simulink model "SwitchOneIR(1)"  (R2019a)
settings: Solver=FixedStepAuto  StartTime=0.0  StopTime=10.0  RelTol=1e-3
libraries: vexarmcortexlib x23, vexcommonlib x3
settings Model: ExtModeTrigDuration=25  Creator=hsstudent  LastModifiedBy=hsstudent
settings SolverCC: AutoInsertRateTranBlk=on
settings OptimizationCC: EnhancedBackFolding=on  PassReuseOutputArgsAs=Individual arguments  MaxStackSize=64  OptimizeBlockOrder=speed  DifferentSizesBufferReuse=on  OptimizationCustomize=off
settings DebuggingCC: ParameterTunabilityLossMsg=error
settings HardwareCC: ProdBitPerPointer=32  ProdBitPerSizeT=32  ProdBitPerPtrDiffT=32  ProdLargestAtomicInteger=Long  ProdLargestAtomicFloat=Double  ProdWordSize=32  ProdHWDeviceType=ARM Compatible->ARM Cortex
settings SFSimCC: MATLABDynamicMemAlloc=off
settings RTWCC: SystemTargetFile=ert.tlc  HardwareBoard=ARM Cortex-based VEX Microcontroller  TLCOptions="-aInlineSetEventsForThisBaseRateFcn=TLC_FALSE -aSuppressMultiTaskScheduler=TLC_FALSE  -aRateBasedStepFcn=0"  TemplateMakefile=ert_default_tmf  GenerateReport=on  Toolchain=GNU Tools for VEX ARM Cortex  IncludeHyperlinkInReport=on  LaunchReport=on  GenerateTraceInfo=on  GenerateTraceReport=on  GenerateTraceReportSl=on  GenerateTraceReportSf=on  GenerateTraceReportEml=on
settings CodeAppCC: ForceParamTrailComments=on  IgnoreCustomStorageClasses=off  OperatorAnnotations=on  SimulinkDataObjDesc=on  SFDataObjDesc=on  InsertBlockDesc=on

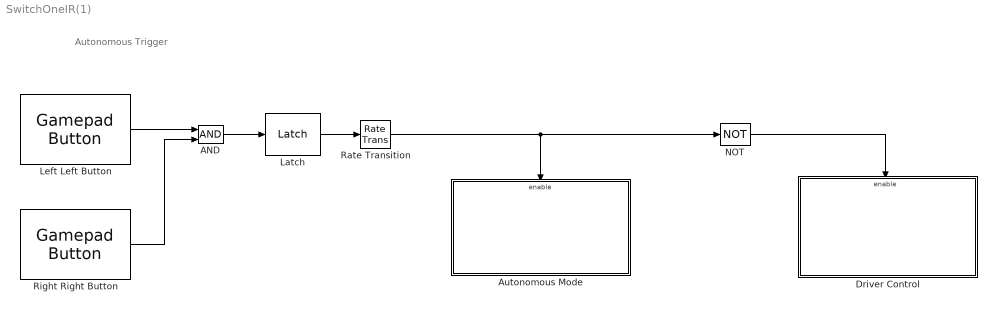
== system SwitchOneIR(1) ==
  note: Autonomous Trigger
  AND : Logic  IconShape=distinctive  AllPortsSameDT=off  OutDataTypeStr=boolean
  Autonomous Mode : Subsystem
  Driver Control : Subsystem  TreatAsAtomicUnit=on
  Latch : vexcommonlib/Latch  output0=off  BlockPlatform=vexarmcortex
      settings: SourceProductName=Simulink Coder Support Package for ARM Cortex-based VEX Microcontroller  SourceProductBaseCode=EC_VEX_MICRO
  Left Left Button : vexarmcortexlib/Gamepad/Gamepad Button  joystick=1  chan=7  button56=Down  button78=Left  SimulationIn=off  SampleTime=0.5
      settings: SourceProductName=Simulink Coder Support Package for ARM Cortex-based VEX Microcontroller  SourceProductBaseCode=EC_VEX_MICRO
  NOT : Logic  Operator=NOT  IconShape=distinctive  AllPortsSameDT=off  OutDataTypeStr=boolean
  Rate Transition : RateTransition
  Right Right Button : vexarmcortexlib/Gamepad/Gamepad Button  joystick=1  chan=8  button56=Down  button78=Right  SimulationIn=off  SampleTime=0.5
      settings: SourceProductName=Simulink Coder Support Package for ARM Cortex-based VEX Microcontroller  SourceProductBaseCode=EC_VEX_MICRO
  wires:
  Rate Transition/1 -> NOT/1, Autonomous Mode/Enable
  AND/1 -> Latch/1
  NOT/1 -> Driver Control/Enable
  Left Left Button/1 -> AND/1
  Latch/1 -> Rate Transition/1
  Right Right Button/1 -> AND/2

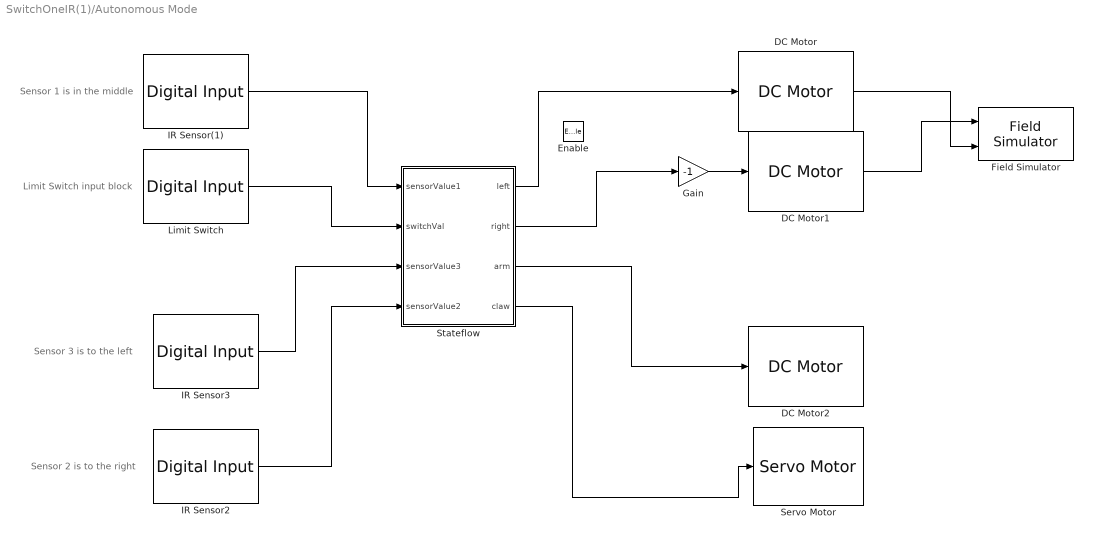
== system SwitchOneIR(1)/Autonomous Mode ==
  note: Sensor 2 is to the right
  note: Sensor 1 is in the middle
  note: Limit Switch input block
  note: Sensor 3 is to the left
  Enable : EnablePort  StatesWhenEnabling=reset
  DC Motor : vexarmcortexlib/Actuators/DC Motor  motor=6  scaleFactor=1/13.5  SimulationOut=on
      settings: SourceProductName=Simulink Coder Support Package for ARM Cortex-based VEX Microcontroller  SourceProductBaseCode=EC_VEX_MICRO
  DC Motor1 : vexarmcortexlib/Actuators/DC Motor  motor=2  scaleFactor=1/13.5  SimulationOut=on
      settings: SourceProductName=Simulink Coder Support Package for ARM Cortex-based VEX Microcontroller  SourceProductBaseCode=EC_VEX_MICRO
  DC Motor2 : vexarmcortexlib/Actuators/DC Motor  motor=9  scaleFactor=1/13.5  SimulationOut=off
      settings: SourceProductName=Simulink Coder Support Package for ARM Cortex-based VEX Microcontroller  SourceProductBaseCode=EC_VEX_MICRO
  Field Simulator : vexcommonlib/Field Simulator  radius=2.5  space=10  range=200  BlockPlatform=vexarmcortex
      settings: SourceProductName=Simulink Coder Support Package for ARM Cortex-based VEX Microcontroller  SourceProductBaseCode=EC_VEX_MICRO
  Gain : Gain  Gain=-1
  IR Sensor(1) : vexarmcortexlib/Sensors/Digital Input  inChan=2  SimulationIn=off  SampleTime=0.05
      settings: SourceProductName=Simulink Coder Support Package for ARM Cortex-based VEX Microcontroller  SourceProductBaseCode=EC_VEX_MICRO
  IR Sensor2 : vexarmcortexlib/Sensors/Digital Input  inChan=8  SimulationIn=off  SampleTime=0.05
      settings: SourceProductName=Simulink Coder Support Package for ARM Cortex-based VEX Microcontroller  SourceProductBaseCode=EC_VEX_MICRO
  IR Sensor3 : vexarmcortexlib/Sensors/Digital Input  inChan=5  SimulationIn=off  SampleTime=0.05
      settings: SourceProductName=Simulink Coder Support Package for ARM Cortex-based VEX Microcontroller  SourceProductBaseCode=EC_VEX_MICRO
  Limit Switch : vexarmcortexlib/Sensors/Digital Input  inChan=6  SimulationIn=off  SampleTime=0.05
      settings: SourceProductName=Simulink Coder Support Package for ARM Cortex-based VEX Microcontroller  SourceProductBaseCode=EC_VEX_MICRO
  Servo Motor : vexarmcortexlib/Actuators/Servo Motor  motor=3  scaleFactor=60/127  SimulationOut=off
      settings: SourceProductName=Simulink Coder Support Package for ARM Cortex-based VEX Microcontroller  SourceProductBaseCode=EC_VEX_MICRO
  Stateflow : Stateflow chart  TreatAsAtomicUnit=on
  wires:
  DC Motor/1 -> Field Simulator/2
  Gain/1 -> DC Motor1/1
  DC Motor1/1 -> Field Simulator/1
  Stateflow/1(left) -> DC Motor/1
  Stateflow/2(right) -> Gain/1
  IR Sensor(1)/1 -> Stateflow/1(sensorValue1)
  Limit Switch/1 -> Stateflow/2(switchVal)
  Stateflow/3(arm) -> DC Motor2/1
  Stateflow/4(claw) -> Servo Motor/1
  IR Sensor2/1 -> Stateflow/4(sensorValue2)
  IR Sensor3/1 -> Stateflow/3(sensorValue3)

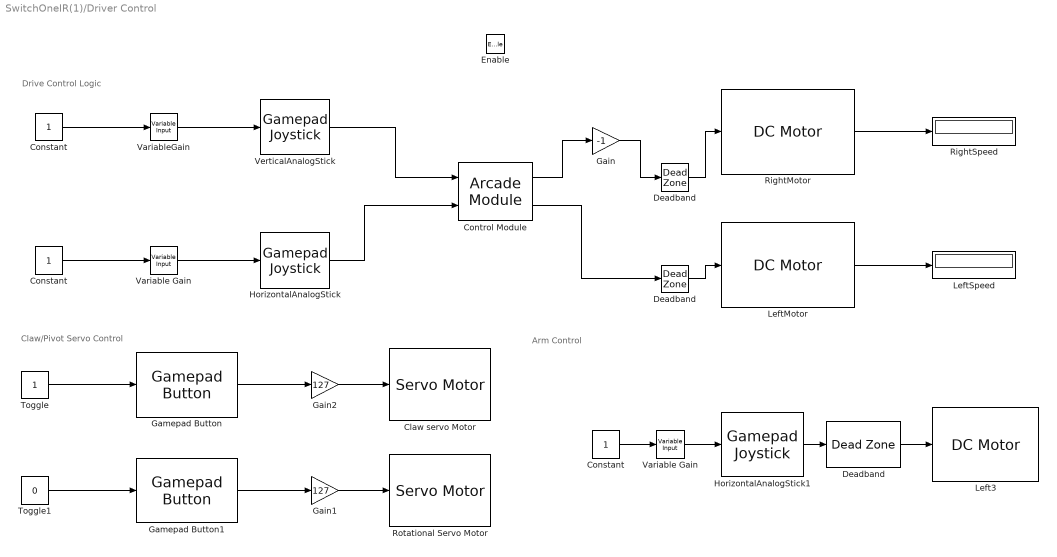
== system SwitchOneIR(1)/Driver Control ==
  note: Claw/Pivot Servo Control
  note: Drive Control Logic
  note: Arm Control
  Enable : EnablePort  StatesWhenEnabling=reset
  "  Deadband " : DeadZone  LowerValue=-30  UpperValue=30  SaturateOnIntegerOverflow=on
  " Constant " : Constant
  " Variable Gain " : vexarmcortexlib/Utilities/Variable Input  low=-127  gain=-68  high=127
      settings: SourceProductName=Simulink Coder Support Package for ARM Cortex-based VEX Microcontroller  SourceProductBaseCode=EC_VEX_MICRO
  Claw servo Motor : vexarmcortexlib/Actuators/Servo Motor  motor=3  scaleFactor=60/127  SimulationOut=off
      settings: SourceProductName=Simulink Coder Support Package for ARM Cortex-based VEX Microcontroller  SourceProductBaseCode=EC_VEX_MICRO
  Constant : Constant
  "Constant " : Constant
  Control Module : vexcommonlib/Arcade Module  BlockPlatform=vexarmcortex
      settings: SourceProductName=Simulink Coder Support Package for ARM Cortex-based VEX Microcontroller  SourceProductBaseCode=EC_VEX_MICRO
  Deadband : DeadZone  SaturateOnIntegerOverflow=on
  "Deadband " : DeadZone  LowerValue=-30  UpperValue=30  SaturateOnIntegerOverflow=on
  Gain : Gain  Gain=-1
  Gain1 : Gain  Gain=127
  Gain2 : Gain  Gain=127
  Gamepad Button : vexarmcortexlib/Gamepad/Gamepad Button  joystick=1  chan=6  button56=Down  button78=Down  SimulationIn=on  SampleTime=0.02
      settings: SourceProductName=Simulink Coder Support Package for ARM Cortex-based VEX Microcontroller  SourceProductBaseCode=EC_VEX_MICRO
  Gamepad Button1 : vexarmcortexlib/Gamepad/Gamepad Button  joystick=1  chan=5  button56=Up  button78=Down  SimulationIn=on  SampleTime=0.02
      settings: SourceProductName=Simulink Coder Support Package for ARM Cortex-based VEX Microcontroller  SourceProductBaseCode=EC_VEX_MICRO
  HorizontalAnalogStick : vexarmcortexlib/Gamepad/Gamepad Joystick  joystick=1  chan=1  SimulationIn=on  SampleTime=0.02
      settings: SourceProductName=Simulink Coder Support Package for ARM Cortex-based VEX Microcontroller  SourceProductBaseCode=EC_VEX_MICRO
  HorizontalAnalogStick1 : vexarmcortexlib/Gamepad/Gamepad Joystick  joystick=1  chan=3  SimulationIn=on  SampleTime=0.02
      settings: SourceProductName=Simulink Coder Support Package for ARM Cortex-based VEX Microcontroller  SourceProductBaseCode=EC_VEX_MICRO
  Left3 : vexarmcortexlib/Actuators/DC Motor  motor=9  scaleFactor=1/13.5  SimulationOut=off
      settings: SourceProductName=Simulink Coder Support Package for ARM Cortex-based VEX Microcontroller  SourceProductBaseCode=EC_VEX_MICRO
  LeftMotor : vexarmcortexlib/Actuators/DC Motor  motor=6  scaleFactor=1/13.5  SimulationOut=on
      settings: SourceProductName=Simulink Coder Support Package for ARM Cortex-based VEX Microcontroller  SourceProductBaseCode=EC_VEX_MICRO
  LeftSpeed : Display
  RightMotor : vexarmcortexlib/Actuators/DC Motor  motor=2  scaleFactor=1/13.5  SimulationOut=on
      settings: SourceProductName=Simulink Coder Support Package for ARM Cortex-based VEX Microcontroller  SourceProductBaseCode=EC_VEX_MICRO
  RightSpeed : Display
  "Rotational Servo Motor " : vexarmcortexlib/Actuators/Servo Motor  motor=8  scaleFactor=60/127  SimulationOut=off
      settings: SourceProductName=Simulink Coder Support Package for ARM Cortex-based VEX Microcontroller  SourceProductBaseCode=EC_VEX_MICRO
  Toggle : Constant
      settings: OpenFcn=|
      | if strcmp('0',get_param(gcb, 'Value'))                        set_param(gcb, 'Value', '1');
      | else
      |             set_param(gcb, 'Value', '0');
      | end
  Toggle1 : Constant  Value=0
      settings: OpenFcn=|
      | if strcmp('0',get_param(gcb, 'Value'))                        set_param(gcb, 'Value', '1');
      | else
      |             set_param(gcb, 'Value', '0');
      | end
  Variable Gain : vexarmcortexlib/Utilities/Variable Input  low=-127  gain=-118.8065  high=127
      settings: SourceProductName=Simulink Coder Support Package for ARM Cortex-based VEX Microcontroller  SourceProductBaseCode=EC_VEX_MICRO
  "VariableGain " : vexarmcortexlib/Utilities/Variable Input  low=-127  gain=0  high=127
      settings: SourceProductName=Simulink Coder Support Package for ARM Cortex-based VEX Microcontroller  SourceProductBaseCode=EC_VEX_MICRO
  VerticalAnalogStick : vexarmcortexlib/Gamepad/Gamepad Joystick  joystick=1  chan=2  SimulationIn=on  SampleTime=0.02
      settings: SourceProductName=Simulink Coder Support Package for ARM Cortex-based VEX Microcontroller  SourceProductBaseCode=EC_VEX_MICRO
  wires:
  Gain2/1 -> Claw servo Motor/1
  Toggle/1 -> Gamepad Button/1
  "Deadband "/1 -> RightMotor/1
  " Variable Gain "/1 -> HorizontalAnalogStick1/1
  " Constant "/1 -> " Variable Gain "/1
  "  Deadband "/1 -> LeftMotor/1
  HorizontalAnalogStick1/1 -> Deadband/1
  Control Module/1 -> Gain/1
  Constant/1 -> "VariableGain "/1
  "VariableGain "/1 -> VerticalAnalogStick/1
  RightMotor/1 -> RightSpeed/1
  Variable Gain/1 -> HorizontalAnalogStick/1
  LeftMotor/1 -> LeftSpeed/1
  Control Module/2 -> "  Deadband "/1
  "Constant "/1 -> Variable Gain/1
  Gamepad Button/1 -> Gain2/1
  Gain/1 -> "Deadband "/1
  VerticalAnalogStick/1 -> Control Module/1
  HorizontalAnalogStick/1 -> Control Module/2
  Deadband/1 -> Left3/1
  Toggle1/1 -> Gamepad Button1/1
  Gain1/1 -> "Rotational Servo Motor "/1
  Gamepad Button1/1 -> Gain1/1

== stateflow chart SwitchOneIR(1)/Autonomous Mode/Stateflow ==
  state Stop
    entry:
    left = 0;
    right= 0;
  state GoForward
    entry:
    left = 100;
    right = 100;
  state GoLeft
    entry:
    left = -50
    right = 50
  note: 
  state Drop
    entry:
    arm = -25;
    left = 0;
    right = 0;
  state GoRight
    entry:
    left = 50
    right = -50
  state ClawDrop
    entry:
    claw = 127;
    left = 0;
    right = 0;
    arm = 0;
  state TowerDetect
    entry:
    left = 0;
    right = 0;
  state Stop2
    entry:
    arm = 0;
    left = 0;
    right = 0;
  (default) -> Stop
  Stop -> GoForward : [sensorValue1 == 0 && sensorValue2 == 1 && sensorValue3 == 1]
  GoForward -> GoLeft [order 1] : [sensorValue1 == 1 && sensorValue2 == 1 && sensorValue3 == 0]
  GoLeft -> GoForward : [sensorValue1 == 0 && sensorValue2 == 1 && sensorValue3 == 1]
  GoForward -> GoRight [order 3] : [sensorValue1 == 1 && sensorValue2 == 0 && sensorValue3 == 1]
  GoForward -> GoRight [order 2] : [sensorValue1 == 0 && sensorValue2 == 1 && sensorValue3 == 1]
  GoForward -> TowerDetect [order 4] : [sensorValue1 == 0 && sensorValue2 == 0 && sensorValue3 == 0]
  GoForward -> TowerDetect [order 5] : [switchVal == 1]
  TowerDetect -> Drop
  Drop -> ClawDrop : after(0.5,sec)
  ClawDrop -> Stop2
  data: left output; right output; sensorValue1 input; switchVal input; arm output; claw output; sensorValue3 input; sensorValue2 input
